simulink model "TestIKEdda2"  (R2020a)
settings: Solver=VariableStepAuto  StartTime=0.0  StopTime=10.0  RelTol=1e-3
values from neighbouring files (symbols this model uses):
  l2 = 0.3    [TestingIkRTR.m]    (also in TestingScriptRTR.m)
undefined symbols (not defined in the file or in its folder): gamma, l1
settings Model: Creator=ja  LastModifiedBy=ja

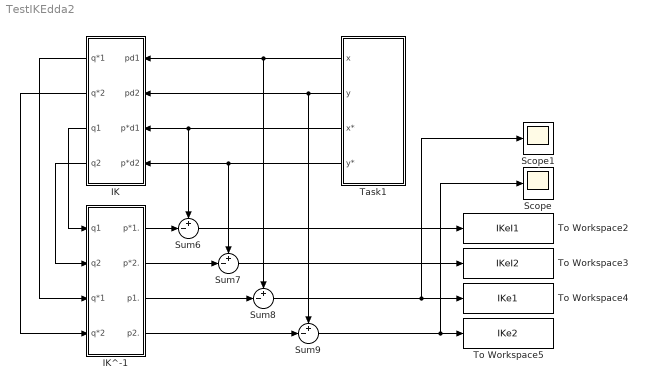
== system TestIKEdda2 ==
  IK : Subsystem
  IK^-1 : Subsystem
  Scope : Scope
  Scope1 : Scope
  Sum{6..9} (4 alike) : Sum  Inputs=+-|
  Task1 : Subsystem
  To Workspace2 : ToWorkspace  VariableName=IKeI1  SampleTime=-1
  To Workspace3 : ToWorkspace  VariableName=IKeI2  SampleTime=-1
  To Workspace4 : ToWorkspace  VariableName=IKe1  SampleTime=-1
  To Workspace5 : ToWorkspace  VariableName=IKe2  SampleTime=-1
  wires:
  Sum9/1 -> Scope/1, To Workspace5/1
  Sum7/1 -> To Workspace3/1
  IK^-1/4(p2.) -> Sum9/2
  Sum6/1 -> To Workspace2/1
  IK^-1/2(p*2.) -> Sum7/2
  Task1/4(y*) -> Sum7/1, IK/4(p*d2)
  Task1/1(x) -> Sum8/1, IK/1(pd1)
  IK/1(q*1) -> IK^-1/3(q*1)
  Task1/2(y) -> IK/2(pd2), Sum9/1
  IK/4(q2) -> IK^-1/2(q2)
  IK/2(q*2) -> IK^-1/4(q*2)
  Sum8/1 -> Scope1/1, To Workspace4/1
  IK^-1/1(p*1.) -> Sum6/2
  IK^-1/3(p1.) -> Sum8/2
  Task1/3(x*) -> Sum6/1, IK/3(p*d1)
  IK/3(q1) -> IK^-1/1(q1)

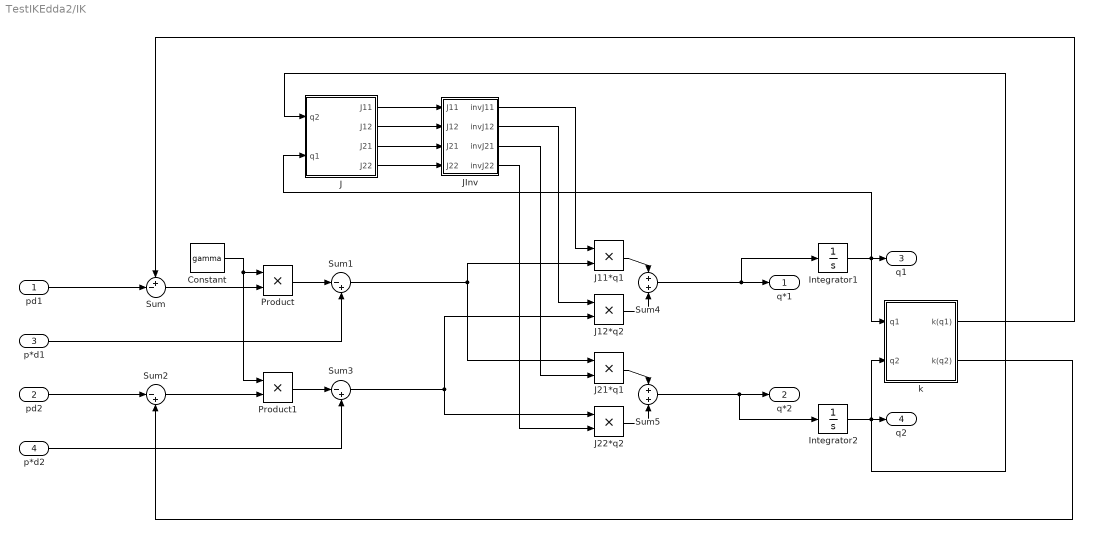
== system TestIKEdda2/IK ==
  pd1 : Inport
  pd2 : Inport  Port=2
  p*d1 : Inport  Port=3
  p*d2 : Inport  Port=4
  Constant : Constant  Value=gamma
  Integrator1 : Integrator  InitialCondition=0.1
  Integrator2 : Integrator  InitialCondition=0.1
  J : Subsystem
  J11*q1 : Product
  J12*q2 : Product
  J21*q1 : Product
  J22*q2 : Product
  JInv : Subsystem
  Product : Product
  Product1 : Product
  Sum : Sum  Inputs=+-|
  Sum1 : Sum  Inputs=|-+
  Sum2 : Sum  Inputs=|-+
  Sum3 : Sum  Inputs=|-+
  Sum4 : Sum
  Sum5 : Sum
  k : Subsystem
  q*1 : Outport
  q*2 : Outport  Port=2
  q1 : Outport  Port=3
  q2 : Outport  Port=4
  wires:
  Sum/1 -> Product/2
  Constant/1 -> Product1/1, Product/1
  pd1/1 -> Sum/2
  Product/1 -> Sum1/1
  p*d1/1 -> Sum1/2
  Product1/1 -> Sum3/1
  Sum2/1 -> Product1/2
  p*d2/1 -> Sum3/2
  J12*q2/1 -> Sum4/2
  J11*q1/1 -> Sum4/1
  J22*q2/1 -> Sum5/2
  J21*q1/1 -> Sum5/1
  Sum4/1 -> Integrator1/1, q*1/1
  Sum5/1 -> Integrator2/1, q*2/1
  Sum3/1 -> J22*q2/1, J12*q2/2
  Sum1/1 -> J11*q1/2, J21*q1/1
  JInv/1(invJ11) -> J11*q1/1
  JInv/2(invJ12) -> J12*q2/1
  JInv/3(invJ21) -> J21*q1/2
  JInv/4(invJ22) -> J22*q2/2
  Integrator1/1 -> J/2(q1), k/1(q1), q1/1
  pd2/1 -> Sum2/1
  Integrator2/1 -> J/1(q2), k/2(q2), q2/1
  J/1(J11) -> JInv/1(J11)
  J/3(J21) -> JInv/3(J21)
  J/2(J12) -> JInv/2(J12)
  J/4(J22) -> JInv/4(J22)
  k/1(k(q1)) -> Sum/1
  k/2(k(q2)) -> Sum2/2

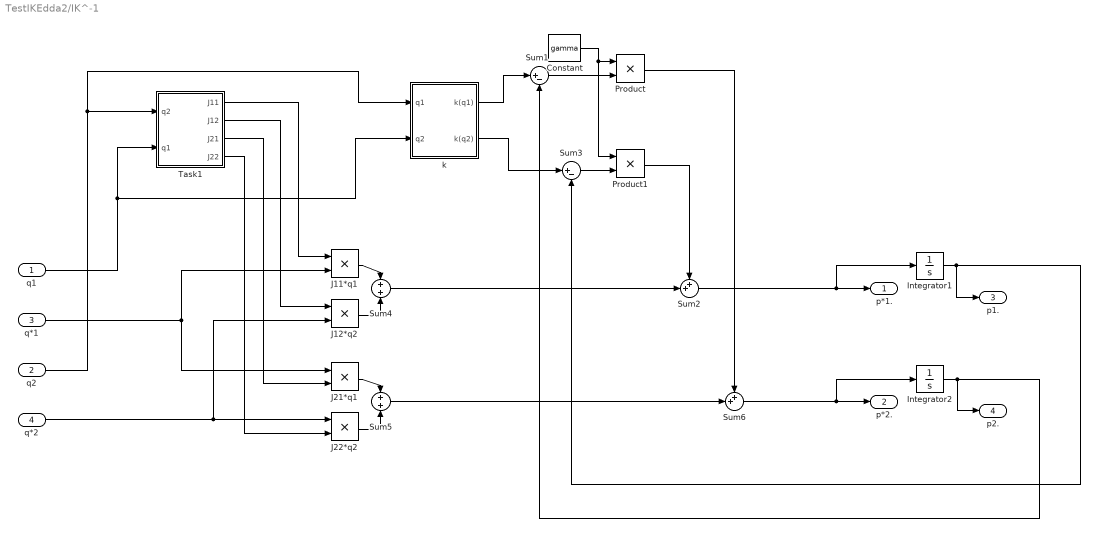
== system TestIKEdda2/IK^-1 ==
  q1 : Inport
  q2 : Inport  Port=2
  q*1 : Inport  Port=3
  q*2 : Inport  Port=4
  Constant : Constant  Value=gamma
  Integrator1 : Integrator  InitialCondition=0.1
  Integrator2 : Integrator  InitialCondition=0.1
  J11*q1 : Product
  J12*q2 : Product
  J21*q1 : Product
  J22*q2 : Product
  Product : Product
  Product1 : Product
  Sum1 : Sum  Inputs=|+-
  Sum2 : Sum  Inputs=++|
  Sum3 : Sum  Inputs=|+-
  Sum4 : Sum
  Sum5 : Sum
  Sum6 : Sum  Inputs=++|
  Task1 : Subsystem
  k : Subsystem
  p*1. : Outport
  p*2. : Outport  Port=2
  p1. : Outport  Port=3
  p2. : Outport  Port=4
  wires:
  Constant/1 -> Product1/1, Product/1
  J12*q2/1 -> Sum4/2
  J11*q1/1 -> Sum4/1
  J22*q2/1 -> Sum5/2
  J21*q1/1 -> Sum5/1
  Task1/1(J11) -> J11*q1/1
  Task1/2(J12) -> J12*q2/1
  Task1/3(J21) -> J21*q1/2
  Task1/4(J22) -> J22*q2/2
  Integrator1/1 -> p1./1, Sum3/2
  Integrator2/1 -> Sum1/2, p2./1
  q1/1 -> k/2(q2), Task1/2(q1)
  q2/1 -> k/1(q1), Task1/1(q2)
  q*1/1 -> J21*q1/1, J11*q1/2
  q*2/1 -> J22*q2/1, J12*q2/2
  Sum1/1 -> Product/2
  k/1(k(q1)) -> Sum1/1
  k/2(k(q2)) -> Sum3/1
  Sum3/1 -> Product1/2
  Sum4/1 -> Sum2/2
  Sum2/1 -> Integrator1/1, p*1./1
  Sum5/1 -> Sum6/2
  Sum6/1 -> Integrator2/1, p*2./1
  Product1/1 -> Sum2/1
  Product/1 -> Sum6/1

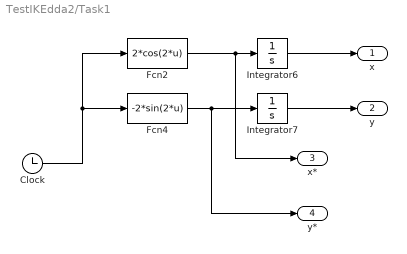
== system TestIKEdda2/Task1 ==
  Clock : Clock
  Fcn2 : Fcn  Expr=2*cos(2*u)
  Fcn4 : Fcn  Expr=-2*sin(2*u)
  Integrator6 : Integrator
  Integrator7 : Integrator  InitialCondition=1
  x : Outport
  y : Outport  Port=2
  x* : Outport  Port=3
  y* : Outport  Port=4
  wires:
  Clock/1 -> Fcn2/1, Fcn4/1
  Integrator6/1 -> x/1
  Integrator7/1 -> y/1
  Fcn2/1 -> x*/1, Integrator6/1
  Fcn4/1 -> y*/1, Integrator7/1

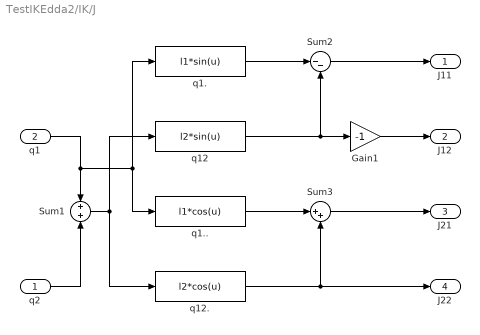
== system TestIKEdda2/IK/J ==
  q2 : Inport
  q1 : Inport  Port=2
  Gain1 : Gain  Gain=-1
  Sum1 : Sum
  Sum2 : Sum  Inputs=|--
  Sum3 : Sum  Inputs=|++
  q1. : Fcn  Expr=l1*sin(u)
  q1.. : Fcn  Expr=l1*cos(u)
  q12 : Fcn  Expr=l2*sin(u)
  q12. : Fcn  Expr=l2*cos(u)
  J11 : Outport
  J12 : Outport  Port=2
  J21 : Outport  Port=3
  J22 : Outport  Port=4
  wires:
  q1/1 -> q1../1, q1./1, Sum1/1
  q2/1 -> Sum1/2
  q1./1 -> Sum2/1
  q12/1 -> Gain1/1, Sum2/2
  Sum2/1 -> J11/1
  Gain1/1 -> J12/1
  q1../1 -> Sum3/1
  q12./1 -> J22/1, Sum3/2
  Sum3/1 -> J21/1
  Sum1/1 -> q12/1, q12./1

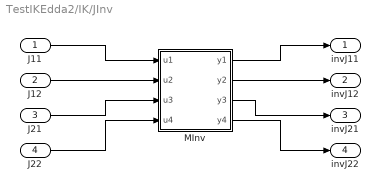
== system TestIKEdda2/IK/JInv ==
  J11 : Inport
  J12 : Inport  Port=2
  J21 : Inport  Port=3
  J22 : Inport  Port=4
  MInv : MATLAB Function  TreatAsAtomicUnit=on
  invJ11 : Outport
  invJ12 : Outport  Port=2
  invJ21 : Outport  Port=3
  invJ22 : Outport  Port=4
  wires:
  J22/1 -> MInv/4(u4)
  J21/1 -> MInv/3(u3)
  J12/1 -> MInv/2(u2)
  J11/1 -> MInv/1(u1)
  MInv/1(y1) -> invJ11/1
  MInv/2(y2) -> invJ12/1
  MInv/3(y3) -> invJ21/1
  MInv/4(y4) -> invJ22/1

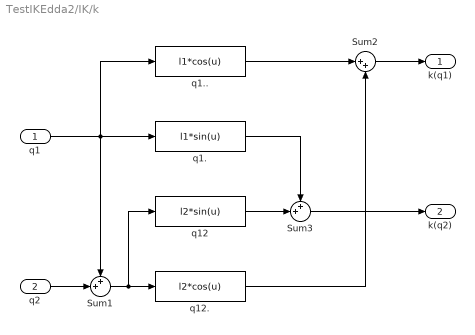
== system TestIKEdda2/IK/k ==
  q1 : Inport
  q2 : Inport  Port=2
  Sum1 : Sum  Inputs=++|
  Sum2 : Sum  Inputs=|++
  Sum3 : Sum  Inputs=++|
  q1. : Fcn  Expr=l1*sin(u)
  q1.. : Fcn  Expr=l1*cos(u)
  q12 : Fcn  Expr=l2*sin(u)
  q12. : Fcn  Expr=l2*cos(u)
  k(q1) : Outport
  k(q2) : Outport  Port=2
  wires:
  q1/1 -> q1../1, q1./1, Sum1/1
  q2/1 -> Sum1/2
  Sum1/1 -> q12/1, q12./1
  q1../1 -> Sum2/1
  Sum3/1 -> k(q2)/1
  Sum2/1 -> k(q1)/1
  q12./1 -> Sum2/2
  q1./1 -> Sum3/1
  q12/1 -> Sum3/2

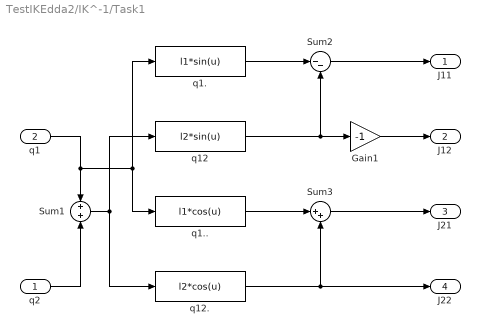
== system TestIKEdda2/IK^-1/Task1 ==
  q2 : Inport
  q1 : Inport  Port=2
  Gain1 : Gain  Gain=-1
  Sum1 : Sum
  Sum2 : Sum  Inputs=|--
  Sum3 : Sum  Inputs=|++
  q1. : Fcn  Expr=l1*sin(u)
  q1.. : Fcn  Expr=l1*cos(u)
  q12 : Fcn  Expr=l2*sin(u)
  q12. : Fcn  Expr=l2*cos(u)
  J11 : Outport
  J12 : Outport  Port=2
  J21 : Outport  Port=3
  J22 : Outport  Port=4
  wires:
  q1/1 -> q1../1, q1./1, Sum1/1
  q2/1 -> Sum1/2
  q1./1 -> Sum2/1
  q12/1 -> Gain1/1, Sum2/2
  Sum2/1 -> J11/1
  Gain1/1 -> J12/1
  q1../1 -> Sum3/1
  q12./1 -> J22/1, Sum3/2
  Sum3/1 -> J21/1
  Sum1/1 -> q12/1, q12./1

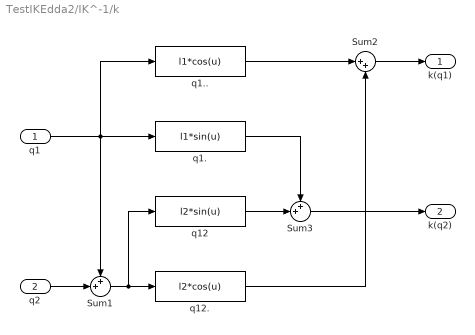
== system TestIKEdda2/IK^-1/k ==
  q1 : Inport
  q2 : Inport  Port=2
  Sum1 : Sum  Inputs=++|
  Sum2 : Sum  Inputs=|++
  Sum3 : Sum  Inputs=++|
  q1. : Fcn  Expr=l1*sin(u)
  q1.. : Fcn  Expr=l1*cos(u)
  q12 : Fcn  Expr=l2*sin(u)
  q12. : Fcn  Expr=l2*cos(u)
  k(q1) : Outport
  k(q2) : Outport  Port=2
  wires:
  q1/1 -> q1../1, q1./1, Sum1/1
  q2/1 -> Sum1/2
  Sum1/1 -> q12/1, q12./1
  q1../1 -> Sum2/1
  Sum3/1 -> k(q2)/1
  Sum2/1 -> k(q1)/1
  q12./1 -> Sum2/2
  q1./1 -> Sum3/1
  q12/1 -> Sum3/2

== matlab function TestIKEdda2/IK/JInv/MInv ==
  data: u1 input; y1 output; u2 input; u3 input; u4 input; y2 output; y3 output; y4 output
function [y1, y2, y3, y4] = c(u1, u2, u3, u4)

y = [u1 u2; u3 u4];
y = inv(y);

y1 = y(1);
y2 = y(2);
y3 = y(3);
y4 = y(4);
